simulink model "NRC_Competition"  (R2025a)
settings: Solver=VariableStepAuto  StartTime=0.0  StopTime=10.0  RelTol=1e-3
settings Model: Creator=jakeo  LastModifiedBy=lukef

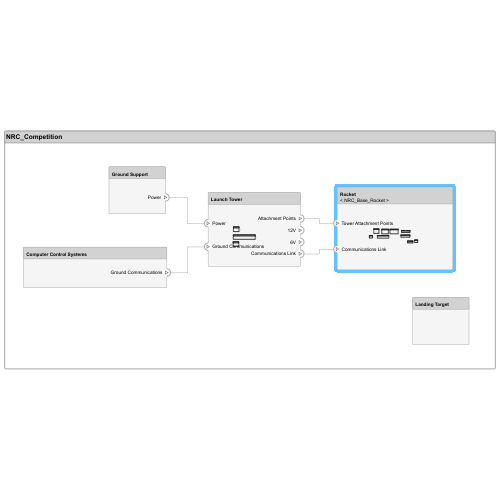
[thumbnail: Simulink's stored preview of the top-level diagram]
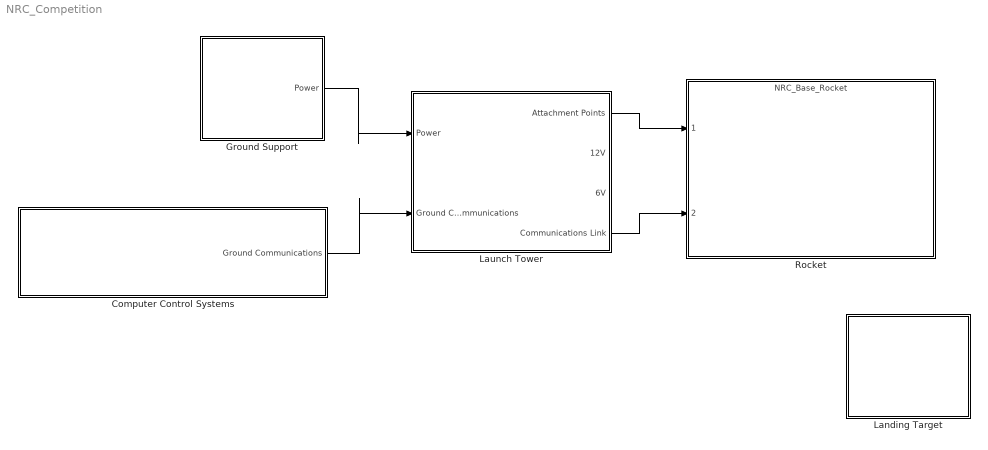
== system NRC_Competition ==
  Computer Control Systems : Subsystem
      settings: PortSchema="{\"entries\":[{\"content\":{\"headerSize\":26,\"margin\":15,\"minimumSpacing\":25,\"sides\":[{\"content\":{},\"type\":\"ConnectorPlacement.EquallySpacedRectSide\",\"uuid\":\"cc45333b-0876-4849-98d5-148de8a70f6b\"},{\"content\":{\"connectorIds\":[\"Out1\"],\"side\":\"RIGHT\"},\"type\":\"ConnectorPlacement.EquallySpacedRectSide\",\"uuid\":\"6d7662cc-0b93-4c22-b72a-22299e415e66\"},{\"content\":{\"side\":\"TOP\"},\"type\":\"ConnectorPlacement.EquallySpacedRectSide\",\"uuid\":\"98fed930-52bb-4e3d-bf56-50c036dee122\"}]},\"type\":\"ConnectorPlacement.EquallySpacedConnector\",\"uuid\":\"dfbe24ca-e965-4cbc-a32c-fe604c746b0d\"}],\"packageUris\":[\"http://schema.mathworks.com/mf0/Connector/R2020b\"],\"version\":\"1.0\"}"
  Ground Support : Subsystem
      settings: PortSchema="{\"entries\":[{\"content\":{\"headerSize\":26,\"margin\":15,\"minimumSpacing\":25,\"sides\":[{\"content\":{},\"type\":\"ConnectorPlacement.EquallySpacedRectSide\",\"uuid\":\"cc45333b-0876-4849-98d5-148de8a70f6b\"},{\"content\":{\"connectorIds\":[\"Out1\"],\"side\":\"RIGHT\"},\"type\":\"ConnectorPlacement.EquallySpacedRectSide\",\"uuid\":\"6d7662cc-0b93-4c22-b72a-22299e415e66\"},{\"content\":{\"side\":\"TOP\"},\"type\":\"ConnectorPlacement.EquallySpacedRectSide\",\"uuid\":\"98fed930-52bb-4e3d-bf56-50c036dee122\"}]},\"type\":\"ConnectorPlacement.EquallySpacedConnector\",\"uuid\":\"dfbe24ca-e965-4cbc-a32c-fe604c746b0d\"}],\"packageUris\":[\"http://schema.mathworks.com/mf0/Connector/R2020b\"],\"version\":\"1.0\"}"
  Landing Target : Subsystem
      settings: PortSchema="{\"entries\":[{\"content\":{\"headerSize\":26,\"margin\":15,\"minimumSpacing\":25,\"sides\":[{\"content\":{},\"type\":\"ConnectorPlacement.EquallySpacedRectSide\",\"uuid\":\"cc45333b-0876-4849-98d5-148de8a70f6b\"},{\"content\":{\"side\":\"RIGHT\"},\"type\":\"ConnectorPlacement.EquallySpacedRectSide\",\"uuid\":\"6d7662cc-0b93-4c22-b72a-22299e415e66\"},{\"content\":{\"side\":\"TOP\"},\"type\":\"ConnectorPlacement.EquallySpacedRectSide\",\"uuid\":\"98fed930-52bb-4e3d-bf56-50c036dee122\"}]},\"type\":\"ConnectorPlacement.EquallySpacedConnector\",\"uuid\":\"dfbe24ca-e965-4cbc-a32c-fe604c746b0d\"}],\"packageUris\":[\"http://schema.mathworks.com/mf0/Connector/R2020b\"],\"version\":\"1.0\"}"
  Launch Tower : Subsystem
      settings: PortSchema="{\"entries\":[{\"content\":{\"headerSize\":26,\"margin\":15,\"minimumSpacing\":25,\"sides\":[{\"content\":{\"connectorIds\":[\"In1\",\"In2\"]},\"type\":\"ConnectorPlacement.EquallySpacedRectSide\",\"uuid\":\"cc45333b-0876-4849-98d5-148de8a70f6b\"},{\"content\":{\"connectorIds\":[\"Out4\",\"Out2\",\"Out3\",\"Out1\"],\"side\":\"RIGHT\"},\"type\":\"ConnectorPlacement.EquallySpacedRectSide\",\"uuid\":\"6d7662cc-0b93-4c22-b72a-22299e415e66\"},{\"content\":{\"side\":\"TOP\"},\"type\":\"ConnectorPlacement.EquallySpacedRectSide\",\"uuid\":\"98fed930-52bb-4e3d-bf56-50c036dee122\"},{\"content\":{\"side\":\"BOTTOM\"},\"type\":\"ConnectorPlacement.EquallySpacedRectSide\",\"uuid\":\"10b6cc0e-d89f-406c-9cc0-d1ac98870dbe\"}]},\"type\":\"ConnectorPlacement.EquallySpacedConnector\",\"uuid\":\"dfbe24ca-e965-4cbc-a32c-fe604c746b0d\"}],\"packageUris\":[\"http://schema.mathworks.com/mf0/Connector/R2020b\"],\"version\":\"1.0\"}"
  Rocket : ModelReference  ModelNameDialog=NRC_Base_Rocket  SimulationMode=Normal  ModelReferenceVersion=2.7
      settings: PortSchema="{\"entries\":[{\"content\":{\"headerSize\":38,\"margin\":15,\"minimumSpacing\":25,\"sides\":[{\"content\":{\"connectorIds\":[\"In1\",\"In2\"]},\"type\":\"ConnectorPlacement.EquallySpacedRectSide\",\"uuid\":\"a6e5da25-d828-4171-97d5-7e7827548b27\"},{\"content\":{\"side\":\"RIGHT\"},\"type\":\"ConnectorPlacement.EquallySpacedRectSide\",\"uuid\":\"0c5b3485-a279-4778-98d7-8b5b9cbe1851\"},{\"content\":{\"side\":\"TOP\"},\"type\":\"ConnectorPlacement.EquallySpacedRectSide\",\"uuid\":\"c965acf9-e7ac-4c11-952e-ee7005e828aa\"}]},\"type\":\"ConnectorPlacement.EquallySpacedConnector\",\"uuid\":\"b06cd9eb-a620-4833-a481-220ed6b8e646\"}],\"packageUris\":[\"http://schema.mathworks.com/mf0/Connector/R2020b\"],\"version\":\"1.0\"}"
  wires:
  Ground Support/1(Power) -> Launch Tower/1(Power)
  Launch Tower/4(Attachment Points) -> Rocket/1
  Launch Tower/1(Communications Link) -> Rocket/2
  Computer Control Systems/1(Ground Communications) -> Launch Tower/2(Ground Communications)

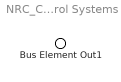
== system NRC_Competition/Computer Control Systems ==
  Bus Element Out1 : Outport  PortName=Ground Communications

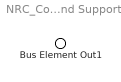
== system NRC_Competition/Ground Support ==
  Bus Element Out1 : Outport  PortName=Power

== system NRC_Competition/Landing Target ==

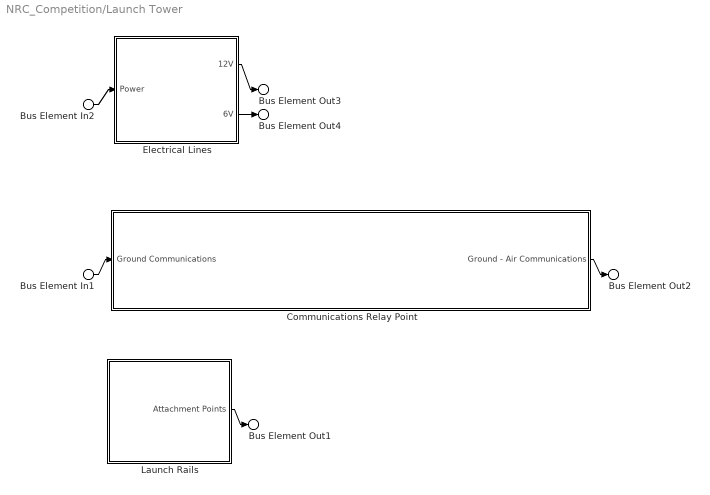
== system NRC_Competition/Launch Tower ==
  Bus Element In2 : Inport  PortName=Power
  Bus Element In1 : Inport  Port=2  PortName=Ground Communications
  Communications Relay Point : Subsystem
      settings: PortSchema="{\"entries\":[{\"content\":{\"headerSize\":26,\"margin\":15,\"minimumSpacing\":25,\"sides\":[{\"content\":{\"connectorIds\":[\"In1\"]},\"type\":\"ConnectorPlacement.EquallySpacedRectSide\",\"uuid\":\"cc45333b-0876-4849-98d5-148de8a70f6b\"},{\"content\":{\"connectorIds\":[\"Out1\"],\"side\":\"RIGHT\"},\"type\":\"ConnectorPlacement.EquallySpacedRectSide\",\"uuid\":\"6d7662cc-0b93-4c22-b72a-22299e415e66\"},{\"content\":{\"side\":\"TOP\"},\"type\":\"ConnectorPlacement.EquallySpacedRectSide\",\"uuid\":\"98fed930-52bb-4e3d-bf56-50c036dee122\"}]},\"type\":\"ConnectorPlacement.EquallySpacedConnector\",\"uuid\":\"dfbe24ca-e965-4cbc-a32c-fe604c746b0d\"}],\"packageUris\":[\"http://schema.mathworks.com/mf0/Connector/R2020b\"],\"version\":\"1.0\"}"
  Electrical Lines : Subsystem
      settings: PortSchema="{\"entries\":[{\"content\":{\"headerSize\":26,\"margin\":15,\"minimumSpacing\":25,\"sides\":[{\"content\":{\"connectorIds\":[\"In1\"]},\"type\":\"ConnectorPlacement.EquallySpacedRectSide\",\"uuid\":\"cc45333b-0876-4849-98d5-148de8a70f6b\"},{\"content\":{\"connectorIds\":[\"Out1\",\"Out2\"],\"side\":\"RIGHT\"},\"type\":\"ConnectorPlacement.EquallySpacedRectSide\",\"uuid\":\"6d7662cc-0b93-4c22-b72a-22299e415e66\"},{\"content\":{\"side\":\"TOP\"},\"type\":\"ConnectorPlacement.EquallySpacedRectSide\",\"uuid\":\"98fed930-52bb-4e3d-bf56-50c036dee122\"}]},\"type\":\"ConnectorPlacement.EquallySpacedConnector\",\"uuid\":\"dfbe24ca-e965-4cbc-a32c-fe604c746b0d\"}],\"packageUris\":[\"http://schema.mathworks.com/mf0/Connector/R2020b\"],\"version\":\"1.0\"}"
  Launch Rails : Subsystem
      settings: PortSchema="{\"entries\":[{\"content\":{\"headerSize\":26,\"margin\":15,\"minimumSpacing\":25,\"sides\":[{\"content\":{},\"type\":\"ConnectorPlacement.EquallySpacedRectSide\",\"uuid\":\"cc45333b-0876-4849-98d5-148de8a70f6b\"},{\"content\":{\"connectorIds\":[\"Out1\"],\"side\":\"RIGHT\"},\"type\":\"ConnectorPlacement.EquallySpacedRectSide\",\"uuid\":\"6d7662cc-0b93-4c22-b72a-22299e415e66\"},{\"content\":{\"side\":\"TOP\"},\"type\":\"ConnectorPlacement.EquallySpacedRectSide\",\"uuid\":\"98fed930-52bb-4e3d-bf56-50c036dee122\"}]},\"type\":\"ConnectorPlacement.EquallySpacedConnector\",\"uuid\":\"dfbe24ca-e965-4cbc-a32c-fe604c746b0d\"}],\"packageUris\":[\"http://schema.mathworks.com/mf0/Connector/R2020b\"],\"version\":\"1.0\"}"
  Bus Element Out2 : Outport  PortName=Communications Link
  Bus Element Out3 : Outport  Port=2  PortName=12V
  Bus Element Out4 : Outport  Port=3  PortName=6V
  Bus Element Out1 : Outport  Port=4  PortName=Attachment Points
  wires:
  Launch Rails/1(Attachment Points) -> Bus Element Out1/1
  Bus Element In1/1 -> Communications Relay Point/1(Ground Communications)
  Communications Relay Point/1(Ground - Air Communications) -> Bus Element Out2/1
  Bus Element In2/1 -> Electrical Lines/1(Power)
  Electrical Lines/1(12V) -> Bus Element Out3/1
  Electrical Lines/2(6V) -> Bus Element Out4/1

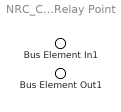
== system NRC_Competition/Launch Tower/Communications Relay Point ==
  Bus Element In1 : Inport  PortName=Ground Communications
  Bus Element Out1 : Outport  PortName=Ground - Air Communications

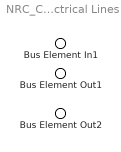
== system NRC_Competition/Launch Tower/Electrical Lines ==
  Bus Element In1 : Inport  PortName=Power
  Bus Element Out1 : Outport  PortName=12V
  Bus Element Out2 : Outport  Port=2  PortName=6V

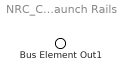
== system NRC_Competition/Launch Tower/Launch Rails ==
  Bus Element Out1 : Outport  PortName=Attachment Points
